simulink model "GUI_V2"  (Simulink 7.7)
settings: Solver=FixedStepDiscrete  SolverMode=SingleTasking  StartTime=0.0  StopTime=60*60*24*365  FixedStep=0.001  RelTol=1e-3
InitFcn:
  | ADB=0;
  | p=1;
  | i1=0;
  | d=0.01;
  | filD=10;
  | 
  | SamT=0.001;
undefined symbols (not defined in the file): Aa1, Bb1, kd, ki, kp, P, R
libraries: simulink x1, Stewart_Gough_LibraryV2 x1, Diamond16AT_UNAL x1
settings Model: Creator=LAB_Mecatronica_16  LastModifiedBy=crist  SimulationMode=external  BufferReuse=off
settings DataIOCC: LimitDataPoints=off
settings OptimizationCC: BlockReduction=off  OptimizeBlockIOStorage=off  BufferReuse=off  ExpressionFolding=off  LocalBlockOutputs=off
settings HardwareCC: ProdIntDivRoundTo=Zero  ProdEndianess=LittleEndian  ProdHWDeviceType=Generic->32-bit x86 compatible
settings RTWCC: SystemTargetFile=xpctarget.tlc  TemplateMakefile=xpc_default_tmf  Description=xPC Target  ProcessScript=xpctarget_make_rtw_hook  RTWCompilerOptimization=On
settings xpcTargetCC: TargetFcnLib=ansi_tfl_table_tmw.mat  TargetFunctionLibrary=XPC_BLAS  FunctionExecutionProfile=off  CodeExecutionProfiling=off  ERTCodeCoverageTool=None  ParMdlRefBuildCompliant=on  CombineSignalStateStructs=off  PortableWordSizes=off  xPCTaskExecutionProfile=off  xPCRL32EventNumber=5000  xPCLoadParamSetFile=off  xPCConcurrentTasks=off  xPCEnableSFAnimation=off

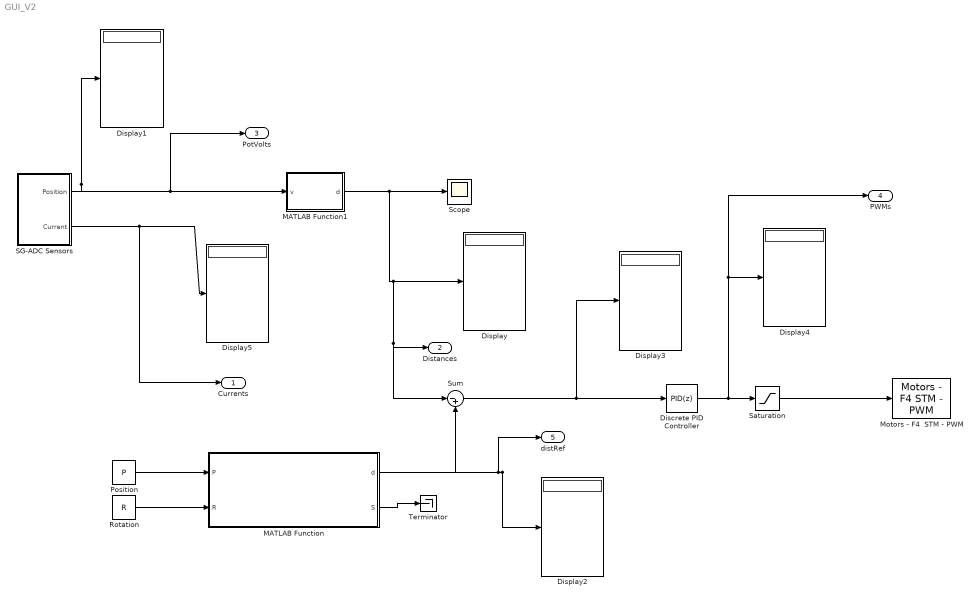
== system GUI_V2 ==
  Discrete PID Controller : simulink/Continuous/PID Controller  SystemSampleTime=-1  Controller=PID  TimeDomain=Discrete-time  SampleTime=1  IntegratorMethod=Forward Euler  FilterMethod=Forward Euler  Form=Parallel  P=kp  I=ki  D=kd  N=100  InitialConditionSource=internal  InitialConditionForIntegrator=0  InitialConditionForFilter=0  ExternalReset=none  LimitOutput=off  UpperSaturationLimit=inf  LowerSaturationLimit=-inf  LinearizeAsGain=off  AntiWindupMode=none  Kb=1  TrackingMode=off  Kt=1  PParamMin=[]  PParamMax=[]  IParamMin=[]  IParamMax=[]  DParamMin=[]  DParamMax=[]  NParamMin=[]  NParamMax=[]  KbParamMin=[]  KbParamMax=[]  KtParamMin=[]  KtParamMax=[]  POutMin=[]  POutMax=[]  IOutMin=[]  IOutMax=[]  DOutMin=[]  DOutMax=[]  NOutMin=[]  NOutMax=[]  KbOutMin=[]  KbOutMax=[]  KtOutMin=[]  KtOutMax=[]  IntegratorOutMin=[]  IntegratorOutMax=[]  FilterOutMin=[]  FilterOutMax=[]  SumOutMin=[]  SumOutMax=[]  SumI1OutMin=[]  SumI1OutMax=[]  SumI2OutMin=[]  SumI2OutMax=[]  SumI3OutMin=[]  SumI3OutMax=[]  SumDOutMin=[]  SumDOutMax=[]  SaturationOutMin=[]  SaturationOutMax=[]  IntegratorContinuousStateAttributes=''  IntegratorStateMustResolveToSignalObject=off  IntegratorRTWStateStorageClass=Auto  FilterContinuousStateAttributes=''  FilterStateMustResolveToSignalObject=off  FilterRTWStateStorageClass=Auto
  Display{,1..5} (6 alike) : Display
      settings: Decimation=3
  MATLAB Function : Stateflow chart  TreatAsAtomicUnit=on
  MATLAB Function1 : Stateflow chart  TreatAsAtomicUnit=on
  Motors - F4  STM - PWM : Stewart_Gough_LibraryV2/SG - Input//Output/Motors - F4  STM - PWM  SystemSampleTime=-1  Satura=80  SamTime=0.001
  Position : Constant  Value=P
  Rotation : Constant  Value=R
  SG-ADC Sensors : Subsystem  AncestorBlock=Stewart_Gough_LibraryV2/SG - Input//Output/SG-ADC Sensors  mask(SG-ADC-Sensors){CutFreq=20, IniSt=[0 0 0 0 0 0], SamTimeADC=0.001}
      mask prompts: CutFreq "Low pass filter - Cutoff frequency (Hz):"; IniSt "Initial States Filter:"; SamTimeADC "Sample Time"
      mask help:
      | ADC from sensors, reading from I/O board diammond 16AT and using a Discrete digital filter to remove measurement noise.
      |
      | OUTPUTS:
      |         [6X1] Measured linear position (mm) for each of the actuators.
      |         [6X1] Measured current (Amp) for each of the actuators.
      mask init:
      | IniStates=[0 IniSt(1)*1.4141;...
      |            0 IniSt(2)*1.4141;...
      |            0 IniSt(3)*1.4141;...
      |            0 IniSt(4)*1.4141;...
      |            0 IniSt(5)*1.4141;...
      |            0 IniSt(6)*1.4141;...                
      |            ];
      | %Filter design
      | n=2;
      | freq=1/SamTimeADC;
      | Wn=CutFreq/(freq/2);          %Sampled to 1kHz and cutof frequency of 20Hz
      | [Aa1,Bb1,Cc1,Dd1]=butter(n,Wn,'low');
      mask Help:
      | ADC from sensors, reading from I/O board diammond 16AT and using a Discrete digital filter to remove measurement noise.
      | 
      | OUTPUTS:
      |         [6X1] Measured linear position (mm) for each of the actuators.
      |         [6X1] Measured current (Amp) for each of the actuators.
      mask TabNameString: Main,Main,Main
  Saturation : Saturate  UpperLimit=90  LowerLimit=-90
  Scope : Scope
      settings: YMin=0  YMax=350
  Sum : Sum  Inputs=|-+
  Terminator : Terminator
  Currents : Outport
  Distances : Outport  Port=2
  PotVolts : Outport  Port=3
  PWMs : Outport  Port=4
  distRef : Outport  Port=5
  wires:
  SG-ADC Sensors/1(Position) -> Display1/1, MATLAB Function1/1(v), PotVolts/1
  Position/1 -> MATLAB Function/1(P)
  Rotation/1 -> MATLAB Function/2(R)
  MATLAB Function/2(S) -> Terminator/1
  SG-ADC Sensors/2(Current) -> Display5/1, Currents/1
  MATLAB Function/1(d) -> Display2/1, Sum/2, distRef/1
  MATLAB Function1/1(d) -> Scope/1, Display/1, Sum/1, Distances/1
  Sum/1 -> Display3/1, Discrete PID Controller/1
  Discrete PID Controller/1 -> Saturation/1, Display4/1, PWMs/1
  Saturation/1 -> Motors - F4  STM - PWM/1

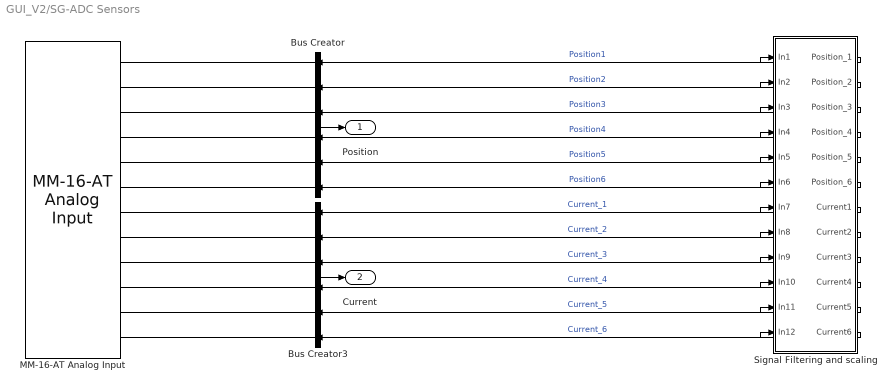
== system GUI_V2/SG-ADC Sensors ==
  Bus Creator : BusCreator  Inputs=6
  Bus Creator3 : BusCreator  Inputs=6
  MM-16-AT Analog Input : Diamond16AT_UNAL/Diamond MM-16-AT/MM-16-AT Analog Input  RequirementInfo={} %GIDa_c23c2098_e60a_40c3_871a_9614e4a60d19  configuration=16 Single-ended  firstChan=1  numChans=12  range=0 to 10V  sampleTime=SamTimeADC  base=300
  Signal Filtering and scaling : Subsystem
  Position : Outport
  Current : Outport  Port=2
  wires:
  Bus Creator3/1 -> Current/1
  Bus Creator/1 -> Position/1
  MM-16-AT Analog Input/6 -> Signal Filtering and scaling/6(In6)
  MM-16-AT Analog Input/12 -> Signal Filtering and scaling/12(In12)
  MM-16-AT Analog Input/11 -> Signal Filtering and scaling/11(In11)
  MM-16-AT Analog Input/10 -> Signal Filtering and scaling/10(In10)
  MM-16-AT Analog Input/9 -> Signal Filtering and scaling/9(In9)
  MM-16-AT Analog Input/8 -> Signal Filtering and scaling/8(In8)
  MM-16-AT Analog Input/7 -> Signal Filtering and scaling/7(In7)
  MM-16-AT Analog Input/5 -> Signal Filtering and scaling/5(In5)
  MM-16-AT Analog Input/4 -> Signal Filtering and scaling/4(In4)
  MM-16-AT Analog Input/3 -> Signal Filtering and scaling/3(In3)
  MM-16-AT Analog Input/2 -> Signal Filtering and scaling/2(In2)
  MM-16-AT Analog Input/1 -> Signal Filtering and scaling/1(In1)
  Signal Filtering and scaling/12(Current6) -> Bus Creator3/6  "Current_6"
  Signal Filtering and scaling/11(Current5) -> Bus Creator3/5  "Current_5"
  Signal Filtering and scaling/10(Current4) -> Bus Creator3/4  "Current_4"
  Signal Filtering and scaling/9(Current3) -> Bus Creator3/3  "Current_3"
  Signal Filtering and scaling/8(Current2) -> Bus Creator3/2  "Current_2"
  Signal Filtering and scaling/7(Current1) -> Bus Creator3/1  "Current_1"
  Signal Filtering and scaling/6(Position_6) -> Bus Creator/6  "Position6"
  Signal Filtering and scaling/5(Position_5) -> Bus Creator/5  "Position5"
  Signal Filtering and scaling/4(Position_4) -> Bus Creator/4  "Position4"
  Signal Filtering and scaling/3(Position_3) -> Bus Creator/3  "Position3"
  Signal Filtering and scaling/2(Position_2) -> Bus Creator/2  "Position2"
  Signal Filtering and scaling/1(Position_1) -> Bus Creator/1  "Position1"

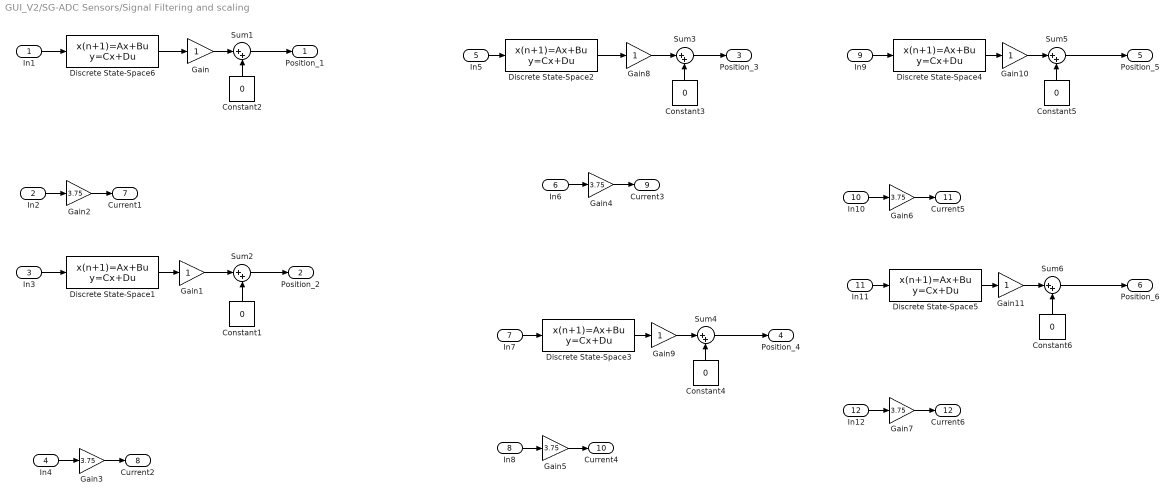
== system GUI_V2/SG-ADC Sensors/Signal Filtering and scaling ==
  In1 : Inport
  In2 : Inport  Port=2
  In3 : Inport  Port=3
  In4 : Inport  Port=4
  In5 : Inport  Port=5
  In6 : Inport  Port=6
  In7 : Inport  Port=7
  In8 : Inport  Port=8
  In9 : Inport  Port=9
  In10 : Inport  Port=10
  In11 : Inport  Port=11
  In12 : Inport  Port=12
  Constant{1..6} (6 alike) : Constant  Value=0
  Discrete State-Space1 : DiscreteStateSpace  A=Aa1  B=Bb1  C=[0 0]  X0=IniStates(2,:)  SampleTime=SamTimeADC
  Discrete State-Space2 : DiscreteStateSpace  A=Aa1  B=Bb1  C=[0 0]  X0=IniStates(3,:)  SampleTime=SamTimeADC
  Discrete State-Space3 : DiscreteStateSpace  A=Aa1  B=Bb1  C=[0 0]  X0=IniStates(4,:)  SampleTime=SamTimeADC
  Discrete State-Space4 : DiscreteStateSpace  A=Aa1  B=Bb1  C=[0 0]  X0=IniStates(5,:)  SampleTime=SamTimeADC
  Discrete State-Space5 : DiscreteStateSpace  A=Aa1  B=Bb1  C=[0 0]  X0=IniStates(5,:)  SampleTime=SamTimeADC
  Discrete State-Space6 : DiscreteStateSpace  A=Aa1  B=Bb1  C=[0 0]  X0=IniStates(1,:)  SampleTime=SamTimeADC
  Gain{,1,8..11} (6 alike) : Gain
  Gain{2..7} (6 alike) : Gain  Gain=3.75
  Sum{1..6} (6 alike) : Sum  Inputs=|++
  Position_1 : Outport
  Position_2 : Outport  Port=2
  Position_3 : Outport  Port=3
  Position_4 : Outport  Port=4
  Position_5 : Outport  Port=5
  Position_6 : Outport  Port=6
  Current1 : Outport  Port=7
  Current2 : Outport  Port=8
  Current3 : Outport  Port=9
  Current4 : Outport  Port=10
  Current5 : Outport  Port=11
  Current6 : Outport  Port=12
  wires:
  In3/1 -> Discrete State-Space1/1
  Discrete State-Space1/1 -> Gain1/1
  Sum2/1 -> Position_2/1
  In5/1 -> Discrete State-Space2/1
  Discrete State-Space2/1 -> Gain8/1
  Sum3/1 -> Position_3/1
  Sum5/1 -> Position_5/1
  Sum6/1 -> Position_6/1
  Discrete State-Space5/1 -> Gain11/1
  In11/1 -> Discrete State-Space5/1
  Discrete State-Space4/1 -> Gain10/1
  In9/1 -> Discrete State-Space4/1
  Sum4/1 -> Position_4/1
  Discrete State-Space3/1 -> Gain9/1
  In7/1 -> Discrete State-Space3/1
  Sum1/1 -> Position_1/1
  Discrete State-Space6/1 -> Gain/1
  In1/1 -> Discrete State-Space6/1
  Constant6/1 -> Sum6/2
  Gain11/1 -> Sum6/1
  Constant5/1 -> Sum5/2
  Gain10/1 -> Sum5/1
  Constant4/1 -> Sum4/2
  Gain9/1 -> Sum4/1
  Constant3/1 -> Sum3/2
  Gain8/1 -> Sum3/1
  Constant1/1 -> Sum2/2
  Gain1/1 -> Sum2/1
  Gain7/1 -> Current6/1
  In12/1 -> Gain7/1
  Gain6/1 -> Current5/1
  In10/1 -> Gain6/1
  Gain5/1 -> Current4/1
  In8/1 -> Gain5/1
  Gain4/1 -> Current3/1
  In6/1 -> Gain4/1
  Gain3/1 -> Current2/1
  In4/1 -> Gain3/1
  Gain2/1 -> Current1/1
  In2/1 -> Gain2/1
  Gain/1 -> Sum1/1
  Constant2/1 -> Sum1/2

== matlab function MATLAB Function1 ==
  data: v input double; d output double
function d = volt2distance(v)

m=[-0.068432671	-0.06935123	-0.06993007	-0.068736142	-0.068432671	-0.068888889]';
b=[0.897373068	0.900514541	0.876083916	0.900243902	0.898741722	0.901]';

d= m.*v + b;

== matlab function MATLAB Function ==
  data: P input double; d output double; R input double; S output double
function [d, S] = inverseKinematics(P, R)
% INVERSEKINEMATICS Inverse kinematics of PRISMMATIC, a SG platform of 
% the Universidad Nacional de Colombia
%
% [d,S] = inverseKinematics(P, aRb) returns the length and direction of 
% each actuator so that the mobile base reaches a desired position P and 
% orientation aRb.
    a = [0.0260    0.1410    0.1149   -0.1149   -0.1410   -0.0260;...
         0.1477   -0.0513   -0.0964   -0.0964   -0.0513    0.1477;...
         0.0380    0.0380    0.0380    0.0380    0.0380    0.0380];
   
    b = [0.0636    0.0869    0.0233   -0.0233   -0.0869   -0.0636;...
         0.0636    0.0233   -0.0869   -0.0869    0.0233    0.0636;...
        -0.0620   -0.0620   -0.0620   -0.0620   -0.0620   -0.0620];

    d = zeros(6,1);
    S = zeros(3,6);
    
    Rz = [cos(R(3)) -sin(R(3)) 0;
          sin(R(3))  cos(R(3)) 0;
                  0          0 1];
    Ry = [cos(R(3)) 0 sin(R(3));
                  0 1         0;
         -sin(R(3)) 0 cos(R(3))];
    Rx = [1         0          0;
          0 cos(R(3)) -sin(R(3));
          0 sin(R(3))  cos(R(3))];
    aRb = Rz*Ry*Rx;

    for i=1:6
        AB = P+aRb*b(:,i)-a(:,i);
        d(i) = norm(AB);
        S(:,i) = AB/d(i);
    end
end
